simulink subsystem "Node_wObserver"  (R2024a)
settings: Solver=VariableStepAuto  StartTime=0.0  StopTime=10.0  RelTol=1e-3
values from neighbouring files (symbols this model uses):
  A = [0 1; 880.87 0]    [main.m]
  B = [0; -9.9453]    [main.m]
  C = [708.27 0]    [main.m]
  K0 = place(A, B, p_desired_tracking)    [main.m]
  Si_x0 = [0 0]'    [main.m]
undefined symbols (not defined in the file or in its folder): closed_loop_dynamics, closed_loop_observer
settings Model: Creator=Stefano  LastModifiedBy=Stefano

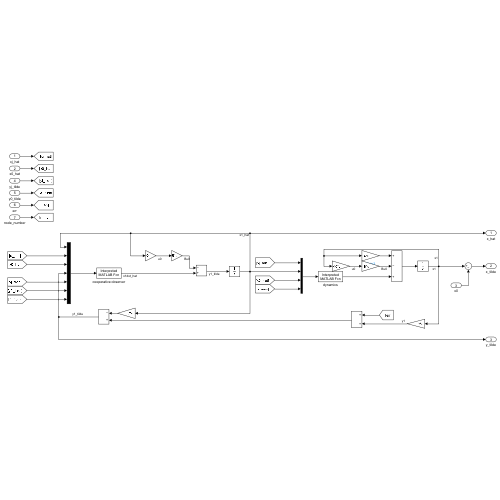
[thumbnail: Simulink's stored preview of the top-level diagram]
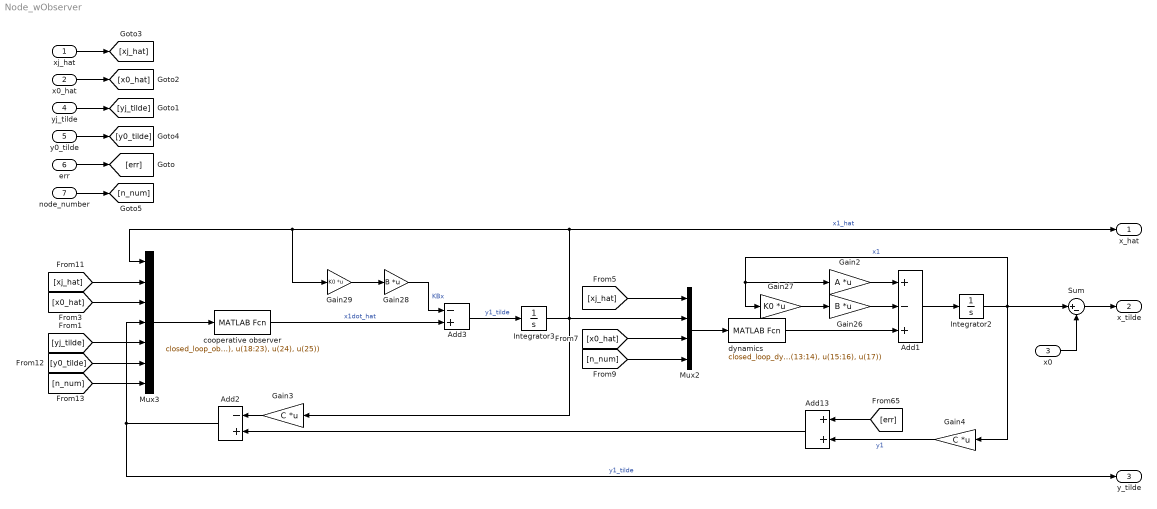
== system Node_wObserver ==
  xj_hat : Inport
  x0_hat : Inport  Port=2
  x0 : Inport  Port=3
  yj_tilde : Inport  Port=4
  y0_tilde : Inport  Port=5
  err : Inport  Port=6
  node_number : Inport  Port=7
  Add1 : Sum  Inputs=+-+
  Add13 : Sum
  Add2 : Sum  Inputs=-+
  Add3 : Sum  Inputs=-+
  Gain2 : Gain  Gain=A  Multiplication=Matrix(K*u)
  Gain26 : Gain  Gain=B  Multiplication=Matrix(K*u)
  Gain27 : Gain  Gain=K0  Multiplication=Matrix(K*u)
  Gain28 : Gain  Gain=B  Multiplication=Matrix(K*u)
  Gain29 : Gain  Gain=K0  Multiplication=Matrix(K*u)
  Gain3 : Gain  Gain=C  Multiplication=Matrix(K*u)
  Gain4 : Gain  Gain=C  Multiplication=Matrix(K*u)
  Integrator2 : Integrator  InitialCondition=Si_x0
  Integrator3 : Integrator  InitialCondition=Si_x0
  Mux2 : Mux
  Mux3 : Mux  Inputs=7
  Sum : Sum  Inputs=|+-
  cooperative observer : MATLABFcn  MATLABFcn=closed_loop_observer(u(1:2), u(3:14), u(15:16), u(17), u(18:23), u(24), u(25))
  dynamics : MATLABFcn  MATLABFcn=closed_loop_dynamics(u(1:12), u(13:14), u(15:16), u(17))
  x_hat : Outport
  x_tilde : Outport  Port=2
  y_tilde : Outport  Port=3
  wires:
  [n_num] -> Mux2/4
  Integrator3/1 -> Mux3/1, Gain29/1, x_hat/1, Mux2/2, Gain3/1  "x1_hat"
  xj_hat/1 -> [xj_hat]
  [xj_hat] -> Mux3/2
  dynamics/1 -> Add1/3
  Add2/1 -> Mux3/4, y_tilde/1  "y1_tilde"
  Mux3/1 -> cooperative observer/1
  Add1/1 -> Integrator2/1
  [x0_hat] -> Mux3/3
  x0_hat/1 -> [x0_hat]
  [x0_hat] -> Mux2/3
  Gain3/1 -> Add2/1
  [yj_tilde] -> Mux3/5
  [xj_hat] -> Mux2/1
  yj_tilde/1 -> [yj_tilde]
  cooperative observer/1 -> Add3/2  "x1dot_hat"
  Gain2/1 -> Add1/1
  Mux2/1 -> dynamics/1
  Gain4/1 -> Add13/2  "y1"
  [y0_tilde] -> Mux3/6
  [n_num] -> Mux3/7
  y0_tilde/1 -> [y0_tilde]
  node_number/1 -> [n_num]
  Sum/1 -> x_tilde/1
  x0/1 -> Sum/2
  Add3/1 -> Integrator3/1  "y1_tilde"
  Gain29/1 -> Gain28/1
  Gain28/1 -> Add3/1  "KBx"
  Add13/1 -> Add2/2
  [err] -> Add13/1
  Integrator2/1 -> Gain4/1, Sum/1, Gain2/1, Gain27/1  "x1"
  Gain26/1 -> Add1/2
  Gain27/1 -> Gain26/1
  err/1 -> [err]
